simulink model "CACC_system_struct"  (Simulink 8.2)
settings: Solver=ode1  SolverMode=SingleTasking  StartTime=0.0  StopTime=inf  FixedStep=0.01  RelTol=1e-3
PreLoadFcn:
  | numd_dvsp = [0.3579 0 -0.3579];
  | dend_dvsp = [1 -1.846 0.8535];
  | simpleacc_param
PostLoadFcn:
  | , if any(exist('dsrtsu_mdlpostloadfcn', 'file') == [2, 3, 6]), try dsrtsu_mdlpostloadfcn('Execute', bdroot); catch fprintf('Error in PostLoadFcn (dsrtsu_mdlpostloadfcn) for model "%s":\n %s\n', bdroot, lasterr); end, end,
undefined symbols (not defined in the file or in its folder): command_mode, max_accel_m_s2, override_enabled, speed_command_m_s, wrench_effort_command
libraries: carma_platform x3, dsrc_transmitter x2, rtitttasklib x2, lightbar x2, srx_platform x1
(part 2 of 4)

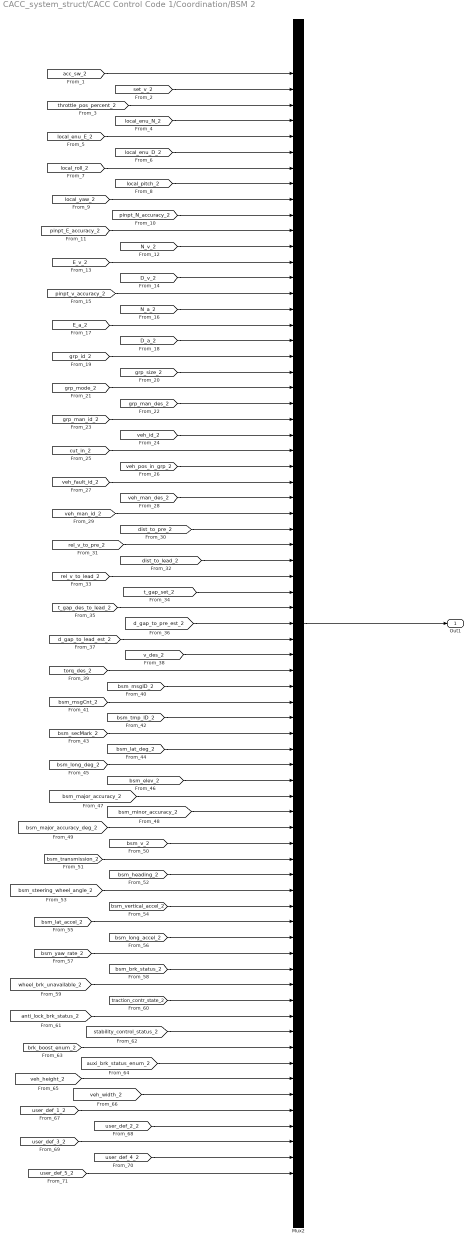
== system CACC_system_struct/CACC Control Code 1/Coordination/BSM 2 ==
  Mux2 : Mux  Inputs=71
  Out1 : Outport
  wires:
  Mux2/1 -> Out1/1
  [user_def_5_2] -> Mux2/71
  [user_def_4_2] -> Mux2/70
  [user_def_3_2] -> Mux2/69
  [user_def_2_2] -> Mux2/68
  [user_def_1_2] -> Mux2/67
  [brk_boost_enum_2] -> Mux2/63
  [auxi_brk_status_enum_2] -> Mux2/64
  [veh_width_2] -> Mux2/66
  [veh_height_2] -> Mux2/65
  [stability_control_status_2] -> Mux2/62
  [anti_lock_brk_status_2] -> Mux2/61
  [traction_contr_state_2] -> Mux2/60
  [wheel_brk_unavailable_2] -> Mux2/59
  [bsm_brk_status_2] -> Mux2/58
  [bsm_yaw_rate_2] -> Mux2/57
  [bsm_long_accel_2] -> Mux2/56
  [bsm_lat_accel_2] -> Mux2/55
  [bsm_vertical_accel_2] -> Mux2/54
  [bsm_steering_wheel_angle_2] -> Mux2/53
  [bsm_heading_2] -> Mux2/52
  [bsm_transmission_2] -> Mux2/51
  [bsm_v_2] -> Mux2/50
  [bsm_major_accuracy_deg_2] -> Mux2/49
  [bsm_minor_accuracy_2] -> Mux2/48
  [bsm_major_accuracy_2] -> Mux2/47
  [bsm_elev_2] -> Mux2/46
  [bsm_long_deg_2] -> Mux2/45
  [bsm_lat_deg_2] -> Mux2/44
  [bsm_secMark_2] -> Mux2/43
  [bsm_tmp_ID_2] -> Mux2/42
  [bsm_msgCnt_2] -> Mux2/41
  [bsm_msgID_2] -> Mux2/40
  [torq_des_2] -> Mux2/39
  [v_des_2] -> Mux2/38
  [d_gap_to_lead_est_2] -> Mux2/37
  [d_gap_to_pre_est_2] -> Mux2/36
  [t_gap_des_to_lead_2] -> Mux2/35
  [t_gap_set_2] -> Mux2/34
  [rel_v_to_lead_2] -> Mux2/33
  [dist_to_lead_2] -> Mux2/32
  [rel_v_to_pre_2] -> Mux2/31
  [dist_to_pre_2] -> Mux2/30
  [veh_man_id_2] -> Mux2/29
  [veh_man_des_2] -> Mux2/28
  [veh_fault_id_2] -> Mux2/27
  [veh_pos_in_grp_2] -> Mux2/26
  [acc_sw_2] -> Mux2/1
  [set_v_2] -> Mux2/2
  [throttle_pos_percent_2] -> Mux2/3
  [local_enu_N_2] -> Mux2/4
  [local_enu_E_2] -> Mux2/5
  [local_enu_D_2] -> Mux2/6
  [local_roll_2] -> Mux2/7
  [local_pitch_2] -> Mux2/8
  [local_yaw_2] -> Mux2/9
  [pinpt_N_accuracy_2] -> Mux2/10
  [pinpt_E_accuracy_2] -> Mux2/11
  [N_v_2] -> Mux2/12
  [E_v_2] -> Mux2/13
  [D_v_2] -> Mux2/14
  [pinpt_v_accuracy_2] -> Mux2/15
  [N_a_2] -> Mux2/16
  [E_a_2] -> Mux2/17
  [D_a_2] -> Mux2/18
  [grp_id_2] -> Mux2/19
  [grp_size_2] -> Mux2/20
  [grp_mode_2] -> Mux2/21
  [grp_man_des_2] -> Mux2/22
  [grp_man_id_2] -> Mux2/23
  [veh_id_2] -> Mux2/24
  [cut_in_2] -> Mux2/25

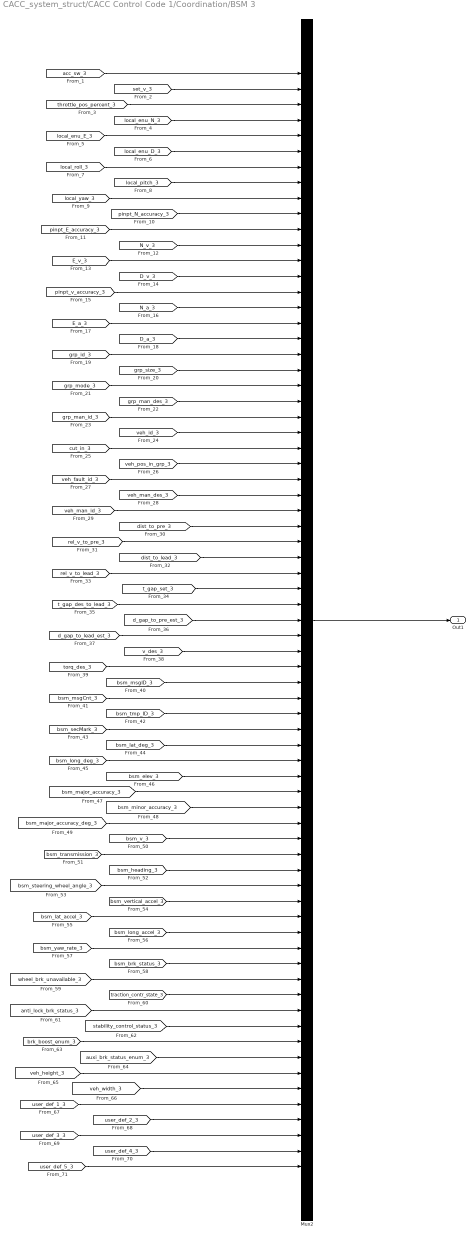
== system CACC_system_struct/CACC Control Code 1/Coordination/BSM 3 ==
  Mux2 : Mux  Inputs=71
  Out1 : Outport
  wires:
  Mux2/1 -> Out1/1
  [user_def_5_3] -> Mux2/71
  [user_def_4_3] -> Mux2/70
  [user_def_3_3] -> Mux2/69
  [user_def_2_3] -> Mux2/68
  [user_def_1_3] -> Mux2/67
  [brk_boost_enum_3] -> Mux2/63
  [auxi_brk_status_enum_3] -> Mux2/64
  [veh_width_3] -> Mux2/66
  [veh_height_3] -> Mux2/65
  [stability_control_status_3] -> Mux2/62
  [anti_lock_brk_status_3] -> Mux2/61
  [traction_contr_state_3] -> Mux2/60
  [wheel_brk_unavailable_3] -> Mux2/59
  [bsm_brk_status_3] -> Mux2/58
  [bsm_yaw_rate_3] -> Mux2/57
  [bsm_long_accel_3] -> Mux2/56
  [bsm_lat_accel_3] -> Mux2/55
  [bsm_vertical_accel_3] -> Mux2/54
  [bsm_steering_wheel_angle_3] -> Mux2/53
  [bsm_heading_3] -> Mux2/52
  [bsm_transmission_3] -> Mux2/51
  [bsm_v_3] -> Mux2/50
  [bsm_major_accuracy_deg_3] -> Mux2/49
  [bsm_minor_accuracy_3] -> Mux2/48
  [bsm_major_accuracy_3] -> Mux2/47
  [bsm_elev_3] -> Mux2/46
  [bsm_long_deg_3] -> Mux2/45
  [bsm_lat_deg_3] -> Mux2/44
  [bsm_secMark_3] -> Mux2/43
  [bsm_tmp_ID_3] -> Mux2/42
  [bsm_msgCnt_3] -> Mux2/41
  [bsm_msgID_3] -> Mux2/40
  [torq_des_3] -> Mux2/39
  [v_des_3] -> Mux2/38
  [d_gap_to_lead_est_3] -> Mux2/37
  [d_gap_to_pre_est_3] -> Mux2/36
  [t_gap_des_to_lead_3] -> Mux2/35
  [t_gap_set_3] -> Mux2/34
  [rel_v_to_lead_3] -> Mux2/33
  [dist_to_lead_3] -> Mux2/32
  [rel_v_to_pre_3] -> Mux2/31
  [dist_to_pre_3] -> Mux2/30
  [veh_man_id_3] -> Mux2/29
  [veh_man_des_3] -> Mux2/28
  [veh_fault_id_3] -> Mux2/27
  [veh_pos_in_grp_3] -> Mux2/26
  [acc_sw_3] -> Mux2/1
  [set_v_3] -> Mux2/2
  [throttle_pos_percent_3] -> Mux2/3
  [local_enu_N_3] -> Mux2/4
  [local_enu_E_3] -> Mux2/5
  [local_enu_D_3] -> Mux2/6
  [local_roll_3] -> Mux2/7
  [local_pitch_3] -> Mux2/8
  [local_yaw_3] -> Mux2/9
  [pinpt_N_accuracy_3] -> Mux2/10
  [pinpt_E_accuracy_3] -> Mux2/11
  [N_v_3] -> Mux2/12
  [E_v_3] -> Mux2/13
  [D_v_3] -> Mux2/14
  [pinpt_v_accuracy_3] -> Mux2/15
  [N_a_3] -> Mux2/16
  [E_a_3] -> Mux2/17
  [D_a_3] -> Mux2/18
  [grp_id_3] -> Mux2/19
  [grp_size_3] -> Mux2/20
  [grp_mode_3] -> Mux2/21
  [grp_man_des_3] -> Mux2/22
  [grp_man_id_3] -> Mux2/23
  [veh_id_3] -> Mux2/24
  [cut_in_3] -> Mux2/25

== system CACC_system_struct/CACC Control Code 1/Coordination/BSM 4 ==
  Mux2 : Mux  Inputs=71
  Out1 : Outport
  wires:
  Mux2/1 -> Out1/1
  [user_def_5_4] -> Mux2/71
  [user_def_4_4] -> Mux2/70
  [user_def_3_4] -> Mux2/69
  [user_def_2_4] -> Mux2/68
  [user_def_1_4] -> Mux2/67
  [brk_boost_enum_4] -> Mux2/63
  [auxi_brk_status_enum_4] -> Mux2/64
  [veh_width_4] -> Mux2/66
  [veh_height_4] -> Mux2/65
  [stability_control_status_4] -> Mux2/62
  [anti_lock_brk_status_4] -> Mux2/61
  [traction_contr_state_4] -> Mux2/60
  [wheel_brk_unavailable_4] -> Mux2/59
  [bsm_brk_status_4] -> Mux2/58
  [bsm_yaw_rate_4] -> Mux2/57
  [bsm_long_accel_4] -> Mux2/56
  [bsm_lat_accel_4] -> Mux2/55
  [bsm_vertical_accel_4] -> Mux2/54
  [bsm_steering_wheel_angle_4] -> Mux2/53
  [bsm_heading_4] -> Mux2/52
  [bsm_transmission_4] -> Mux2/51
  [bsm_v_4] -> Mux2/50
  [bsm_major_accuracy_deg_4] -> Mux2/49
  [bsm_minor_accuracy_4] -> Mux2/48
  [bsm_major_accuracy_4] -> Mux2/47
  [bsm_elev_4] -> Mux2/46
  [bsm_long_deg_4] -> Mux2/45
  [bsm_lat_deg_4] -> Mux2/44
  [bsm_secMark_4] -> Mux2/43
  [bsm_tmp_ID_4] -> Mux2/42
  [bsm_msgCnt_4] -> Mux2/41
  [bsm_msgID_4] -> Mux2/40
  [torq_des_4] -> Mux2/39
  [v_des_4] -> Mux2/38
  [d_gap_to_lead_est_4] -> Mux2/37
  [d_gap_to_pre_est_4] -> Mux2/36
  [t_gap_des_to_lead_4] -> Mux2/35
  [t_gap_set_4] -> Mux2/34
  [rel_v_to_lead_4] -> Mux2/33
  [dist_to_lead_4] -> Mux2/32
  [rel_v_to_pre_4] -> Mux2/31
  [dist_to_pre_4] -> Mux2/30
  [veh_man_id_4] -> Mux2/29
  [veh_man_des_4] -> Mux2/28
  [veh_fault_id_4] -> Mux2/27
  [veh_pos_in_grp_4] -> Mux2/26
  [acc_sw_4] -> Mux2/1
  [set_v_4] -> Mux2/2
  [throttle_pos_percent_4] -> Mux2/3
  [local_enu_N_4] -> Mux2/4
  [local_enu_E_4] -> Mux2/5
  [local_enu_D_4] -> Mux2/6
  [local_roll_4] -> Mux2/7
  [local_pitch_4] -> Mux2/8
  [local_yaw_4] -> Mux2/9
  [pinpt_N_accuracy_4] -> Mux2/10
  [pinpt_E_accuracy_4] -> Mux2/11
  [N_v_4] -> Mux2/12
  [E_v_4] -> Mux2/13
  [D_v_4] -> Mux2/14
  [pinpt_v_accuracy_4] -> Mux2/15
  [N_a_4] -> Mux2/16
  [E_a_4] -> Mux2/17
  [D_a_4] -> Mux2/18
  [grp_id_4] -> Mux2/19
  [grp_size_4] -> Mux2/20
  [grp_mode_4] -> Mux2/21
  [grp_man_des_4] -> Mux2/22
  [grp_man_id_4] -> Mux2/23
  [veh_id_4] -> Mux2/24
  [cut_in_4] -> Mux2/25

== system CACC_system_struct/CACC Control Code 1/Coordination/BSM 5 ==
  Mux2 : Mux  Inputs=71
  Out1 : Outport
  wires:
  Mux2/1 -> Out1/1
  [user_def_5_5] -> Mux2/71
  [user_def_4_5] -> Mux2/70
  [user_def_3_5] -> Mux2/69
  [user_def_2_5] -> Mux2/68
  [user_def_1_5] -> Mux2/67
  [brk_boost_enum_5] -> Mux2/63
  [auxi_brk_status_enum_5] -> Mux2/64
  [veh_width_5] -> Mux2/66
  [veh_height_5] -> Mux2/65
  [stability_control_status_5] -> Mux2/62
  [anti_lock_brk_status_5] -> Mux2/61
  [traction_contr_state_5] -> Mux2/60
  [wheel_brk_unavailable_5] -> Mux2/59
  [bsm_brk_status_5] -> Mux2/58
  [bsm_yaw_rate_5] -> Mux2/57
  [bsm_long_accel_5] -> Mux2/56
  [bsm_lat_accel_5] -> Mux2/55
  [bsm_vertical_accel_5] -> Mux2/54
  [bsm_steering_wheel_angle_5] -> Mux2/53
  [bsm_heading_5] -> Mux2/52
  [bsm_transmission_5] -> Mux2/51
  [bsm_v_5] -> Mux2/50
  [bsm_major_accuracy_deg_5] -> Mux2/49
  [bsm_minor_accuracy_5] -> Mux2/48
  [bsm_major_accuracy_5] -> Mux2/47
  [bsm_elev_5] -> Mux2/46
  [bsm_long_deg_5] -> Mux2/45
  [bsm_lat_deg_5] -> Mux2/44
  [bsm_secMark_5] -> Mux2/43
  [bsm_tmp_ID_5] -> Mux2/42
  [bsm_msgCnt_5] -> Mux2/41
  [bsm_msgID_5] -> Mux2/40
  [torq_des_5] -> Mux2/39
  [v_des_5] -> Mux2/38
  [d_gap_to_lead_est_5] -> Mux2/37
  [d_gap_to_pre_est_5] -> Mux2/36
  [t_gap_des_to_lead_5] -> Mux2/35
  [t_gap_set_5] -> Mux2/34
  [rel_v_to_lead_5] -> Mux2/33
  [dist_to_lead_5] -> Mux2/32
  [rel_v_to_pre_5] -> Mux2/31
  [dist_to_pre_5] -> Mux2/30
  [veh_man_id_5] -> Mux2/29
  [veh_man_des_5] -> Mux2/28
  [veh_fault_id_5] -> Mux2/27
  [veh_pos_in_grp_5] -> Mux2/26
  [acc_sw_5] -> Mux2/1
  [set_v_5] -> Mux2/2
  [throttle_pos_percent_5] -> Mux2/3
  [local_enu_N_5] -> Mux2/4
  [local_enu_E_5] -> Mux2/5
  [local_enu_D_5] -> Mux2/6
  [local_roll_5] -> Mux2/7
  [local_pitch_5] -> Mux2/8
  [local_yaw_5] -> Mux2/9
  [pinpt_N_accuracy_5] -> Mux2/10
  [pinpt_E_accuracy_5] -> Mux2/11
  [N_v_5] -> Mux2/12
  [E_v_5] -> Mux2/13
  [D_v_5] -> Mux2/14
  [pinpt_v_accuracy_5] -> Mux2/15
  [N_a_5] -> Mux2/16
  [E_a_5] -> Mux2/17
  [D_a_5] -> Mux2/18
  [grp_id_5] -> Mux2/19
  [grp_size_5] -> Mux2/20
  [grp_mode_5] -> Mux2/21
  [grp_man_des_5] -> Mux2/22
  [grp_man_id_5] -> Mux2/23
  [veh_id_5] -> Mux2/24
  [cut_in_5] -> Mux2/25

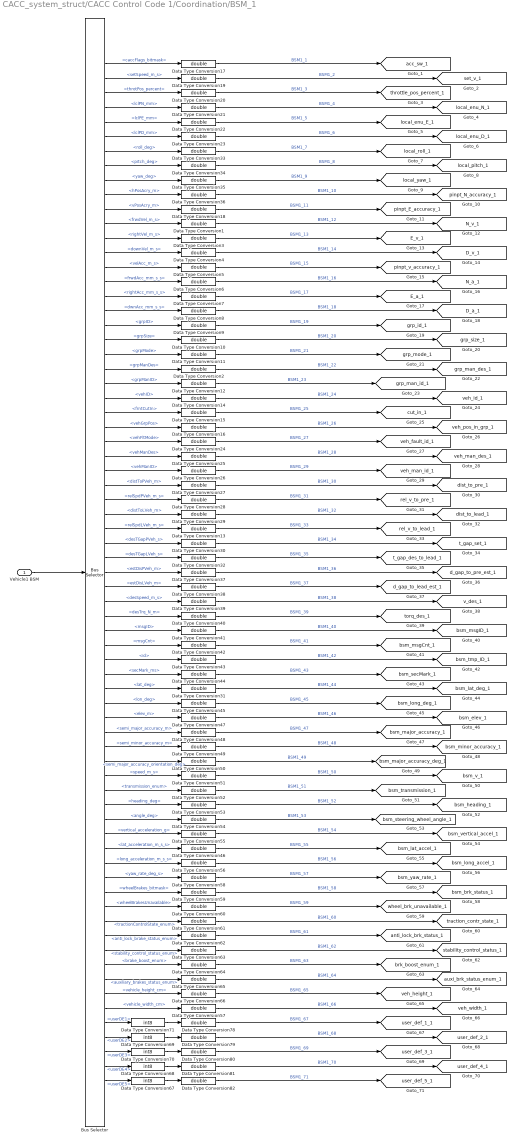
== system CACC_system_struct/CACC Control Code 1/Coordination/BSM_1 ==
  Vehicle1 BSM : Inport
  Bus Selector : BusSelector  OutputSignals=caccFlags_bitmask,setSpeed_m_s,throtPos_percent,lclPN_mm,lclPE_mm,lclPD_mm,roll_deg,pitch_deg,yaw_deg,hPosAcry_m,vPosAcry_m,frwdVel_m_s,rightVel_m_s,downVel_m_s,velAcc_m_s,frwdAcc_mm_s_s,rightAcc_mm_s_s,dwnAcc_mm_s_s,grpID,grpSize,grpMode,grpManDes,grpManID,vehID,frntCutIn,vehGrpPos,vehFltMode,vehManDes,vehManID,distToPVeh_m,relSpdPVeh_m_s,distToLVeh_m,relSpdLVeh_m_s,desTGapPVeh_s,desTGapLVeh_s,estDisPVeh_m,estDisLVeh_m,desSpeed_m_s,desTrq_N_m,msgID,msgCnt,id,secMark_ms,lat_deg,lon_deg,elev_m,semi_major_accuracy_m,semi_minor_accuracy_m,semi_major_accuracy_orientation_deg,speed_m_s,transmission_enum,heading_deg,angle_deg,vertical_acceleration_g,lat_acceleration_m_s_s,long_acceleration_m_s_s,yaw_rate_deg_s,wheelBrakes_bitmask,wheelBrakesUnavailable,tractionControlState_enum,anti_lock_brake_status_enum,stability_control_status_enum,brake_boost_enum,auxiliary_brakes_status_enum,vehicle_height_cm,vehicle_width_cm,userDE1,userDE2,userDE3,userDE4,userDE5
  Data Type Conversion{1..66,78..82} (71 alike) : DataTypeConversion  OutMin=[0]  OutMax=[5]  OutDataTypeStr=double
  Data Type Conversion{67..71} (5 alike) : DataTypeConversion  OutMin=[-128]  OutMax=[127]  OutDataTypeStr=int8  ConvertRealWorld=Stored Integer (SI)
  tag scope: D_a_1=global, D_v_1=global, E_a_1=global, E_v_1=global, N_a_1=global, N_v_1=global, acc_sw_1=global, anti_lock_brk_status_1=global, auxi_brk_status_enum_1=global, brk_boost_enum_1=global, bsm_brk_status_1=global, bsm_elev_1=global, bsm_heading_1=global, bsm_lat_accel_1=global, bsm_lat_deg_1=global, bsm_long_accel_1=global, bsm_long_deg_1=global, bsm_major_accuracy_1=global, bsm_major_accuracy_deg_1=global, bsm_minor_accuracy_1=global, bsm_msgCnt_1=global, bsm_msgID_1=global, bsm_secMark_1=global, bsm_steering_wheel_angle_1=global, bsm_tmp_ID_1=global, bsm_transmission_1=global, bsm_v_1=global, bsm_vertical_accel_1=global, bsm_yaw_rate_1=global, cut_in_1=global, d_gap_to_lead_est_1=global, d_gap_to_pre_est_1=global, dist_to_lead_1=global, dist_to_pre_1=global, grp_id_1=global, grp_man_des_1=global, grp_man_id_1=global, grp_mode_1=global, grp_size_1=global, local_enu_D_1=global, local_enu_E_1=global, local_enu_N_1=global, local_pitch_1=global, local_roll_1=global, local_yaw_1=global, pinpt_E_accuracy_1=global, pinpt_N_accuracy_1=global, pinpt_v_accuracy_1=global, rel_v_to_lead_1=global, rel_v_to_pre_1=global, set_v_1=global, stability_control_status_1=global, t_gap_des_to_lead_1=global, t_gap_set_1=global, throttle_pos_percent_1=global, torq_des_1=global, traction_contr_state_1=global, user_def_1_1=global, user_def_2_1=global, user_def_3_1=global, user_def_4_1=global, user_def_5_1=global, v_des_1=global, veh_fault_id_1=global, veh_height_1=global, veh_id_1=global, veh_man_des_1=global, veh_man_id_1=global, veh_pos_in_grp_1=global, veh_width_1=global, wheel_brk_unavailable_1=global
  wires:
  Vehicle1 BSM/1 -> Bus Selector/1
  Bus Selector/34 -> Data Type Conversion30/1  "<desTGapPVeh_s>"
  Bus Selector/33 -> Data Type Conversion13/1  "<relSpdLVeh_m_s>"
  Bus Selector/2 -> Data Type Conversion19/1  "<setSpeed_m_s>"
  Bus Selector/1 -> Data Type Conversion17/1  "<caccFlags_bitmask>"
  Bus Selector/7 -> Data Type Conversion33/1  "<roll_deg>"
  Bus Selector/3 -> Data Type Conversion20/1  "<throtPos_percent>"
  Bus Selector/9 -> Data Type Conversion35/1  "<yaw_deg>"
  Bus Selector/8 -> Data Type Conversion34/1  "<pitch_deg>"
  Bus Selector/11 -> Data Type Conversion18/1  "<vPosAcry_m>"
  Bus Selector/10 -> Data Type Conversion36/1  "<hPosAcry_m>"
  Bus Selector/13 -> Data Type Conversion3/1  "<rightVel_m_s>"
  Bus Selector/12 -> Data Type Conversion1/1  "<frwdVel_m_s>"
  Bus Selector/15 -> Data Type Conversion5/1  "<velAcc_m_s>"
  Bus Selector/14 -> Data Type Conversion4/1  "<downVel_m_s>"
  Bus Selector/17 -> Data Type Conversion7/1  "<rightAcc_mm_s_s>"
  Bus Selector/16 -> Data Type Conversion6/1  "<frwdAcc_mm_s_s>"
  Bus Selector/19 -> Data Type Conversion9/1  "<grpID>"
  Bus Selector/18 -> Data Type Conversion8/1  "<dwnAcc_mm_s_s>"
  Bus Selector/21 -> Data Type Conversion11/1  "<grpMode>"
  Bus Selector/20 -> Data Type Conversion10/1  "<grpSize>"
  Bus Selector/22 -> Data Type Conversion2/1  "<grpManDes>"
  Bus Selector/25 -> Data Type Conversion15/1  "<frntCutIn>"
  Bus Selector/24 -> Data Type Conversion14/1  "<vehID>"
  Bus Selector/27 -> Data Type Conversion24/1  "<vehFltMode>"
  Bus Selector/26 -> Data Type Conversion16/1  "<vehGrpPos>"
  Bus Selector/30 -> Data Type Conversion27/1  "<distToPVeh_m>"
  Bus Selector/29 -> Data Type Conversion26/1  "<vehManID>"
  Bus Selector/32 -> Data Type Conversion29/1  "<distToLVeh_m>"
  Bus Selector/36 -> Data Type Conversion37/1  "<estDisPVeh_m>"
  Bus Selector/35 -> Data Type Conversion32/1  "<desTGapLVeh_s>"
  Bus Selector/38 -> Data Type Conversion39/1  "<desSpeed_m_s>"
  Bus Selector/37 -> Data Type Conversion38/1  "<estDisLVeh_m>"
  Bus Selector/40 -> Data Type Conversion41/1  "<msgID>"
  Bus Selector/39 -> Data Type Conversion40/1  "<desTrq_N_m>"
  Bus Selector/42 -> Data Type Conversion43/1  "<id>"
  Bus Selector/41 -> Data Type Conversion42/1  "<msgCnt>"
  Bus Selector/44 -> Data Type Conversion31/1  "<lat_deg>"
  Bus Selector/43 -> Data Type Conversion44/1  "<secMark_ms>"
  Bus Selector/46 -> Data Type Conversion47/1  "<elev_m>"
  Bus Selector/45 -> Data Type Conversion45/1  "<lon_deg>"
  Bus Selector/48 -> Data Type Conversion49/1  "<semi_minor_accuracy_m>"
  Bus Selector/47 -> Data Type Conversion48/1  "<semi_major_accuracy_m>"
  Bus Selector/50 -> Data Type Conversion51/1  "<speed_m_s>"
  Bus Selector/49 -> Data Type Conversion50/1  "<semi_major_accuracy_orientation_deg>"
  Bus Selector/52 -> Data Type Conversion53/1  "<heading_deg>"
  Bus Selector/51 -> Data Type Conversion52/1  "<transmission_enum>"
  Bus Selector/54 -> Data Type Conversion55/1  "<vertical_acceleration_g>"
  Bus Selector/53 -> Data Type Conversion54/1  "<angle_deg>"
  Bus Selector/56 -> Data Type Conversion56/1  "<long_acceleration_m_s_s>"
  Bus Selector/55 -> Data Type Conversion46/1  "<lat_acceleration_m_s_s>"
  Bus Selector/58 -> Data Type Conversion59/1  "<wheelBrakes_bitmask>"
  Bus Selector/57 -> Data Type Conversion58/1  "<yaw_rate_deg_s>"
  Bus Selector/60 -> Data Type Conversion61/1  "<tractionControlState_enum>"
  Bus Selector/59 -> Data Type Conversion60/1  "<wheelBrakesUnavailable>"
  Bus Selector/62 -> Data Type Conversion63/1  "<stability_control_status_enum>"
  Bus Selector/61 -> Data Type Conversion62/1  "<anti_lock_brake_status_enum>"
  Bus Selector/64 -> Data Type Conversion65/1  "<auxiliary_brakes_status_enum>"
  Bus Selector/63 -> Data Type Conversion64/1  "<brake_boost_enum>"
  Bus Selector/66 -> Data Type Conversion57/1  "<vehicle_width_cm>"
  Bus Selector/65 -> Data Type Conversion66/1  "<vehicle_height_cm>"
  Bus Selector/4 -> Data Type Conversion21/1  "<lclPN_mm>"
  Bus Selector/5 -> Data Type Conversion22/1  "<lclPE_mm>"
  Bus Selector/6 -> Data Type Conversion23/1  "<lclPD_mm>"
  Bus Selector/23 -> Data Type Conversion12/1  "<grpManID>"
  Bus Selector/28 -> Data Type Conversion25/1  "<vehManDes>"
  Bus Selector/31 -> Data Type Conversion28/1  "<relSpdPVeh_m_s>"
  Bus Selector/67 -> Data Type Conversion71/1  "<userDE1>"
  Bus Selector/68 -> Data Type Conversion69/1  "<userDE2>"
  Bus Selector/69 -> Data Type Conversion70/1  "<userDE3>"
  Bus Selector/70 -> Data Type Conversion68/1  "<userDE4>"
  Bus Selector/71 -> Data Type Conversion67/1  "<userDE5>"
  Data Type Conversion25/1 -> [veh_man_des_1]  "BSM1_28"
  Data Type Conversion17/1 -> [acc_sw_1]  "BSM1_1"
  Data Type Conversion52/1 -> [bsm_transmission_1]  "BSM1_51"
  Data Type Conversion1/1 -> [N_v_1]  "BSM1_12"
  Data Type Conversion11/1 -> [grp_mode_1]  "BSM1_21"
  Data Type Conversion13/1 -> [rel_v_to_lead_1]  "BSM1_33"
  Data Type Conversion3/1 -> [E_v_1]  "BSM1_13"
  Data Type Conversion56/1 -> [bsm_long_accel_1]  "BSM1_56"
  Data Type Conversion14/1 -> [veh_id_1]  "BSM1_24"
  Data Type Conversion18/1 -> [pinpt_E_accuracy_1]  "BSM1_11"
  Data Type Conversion53/1 -> [bsm_heading_1]  "BSM1_52"
  Data Type Conversion55/1 -> [bsm_vertical_accel_1]  "BSM1_54"
  Data Type Conversion27/1 -> [dist_to_pre_1]  "BSM1_30"
  Data Type Conversion23/1 -> [local_enu_D_1]  "BSM1_6"
  Data Type Conversion21/1 -> [local_enu_N_1]  "BSM1_4"
  Data Type Conversion22/1 -> [local_enu_E_1]  "BSM1_5"
  Data Type Conversion28/1 -> [rel_v_to_pre_1]  "BSM1_31"
  Data Type Conversion12/1 -> [grp_man_id_1]  "BSM1_23"
  Data Type Conversion49/1 -> [bsm_minor_accuracy_1]  "BSM1_48"
  Data Type Conversion24/1 -> [veh_fault_id_1]  "BSM1_27"
  Data Type Conversion26/1 -> [veh_man_id_1]  "BSM1_29"
  Data Type Conversion10/1 -> [grp_size_1]  "BSM1_20"
  Data Type Conversion19/1 -> [set_v_1]  "BSM1_2"
  Data Type Conversion29/1 -> [dist_to_lead_1]  "BSM1_32"
  Data Type Conversion51/1 -> [bsm_v_1]  "BSM1_50"
  Data Type Conversion57/1 -> [veh_width_1]  "BSM1_66"
  Data Type Conversion20/1 -> [throttle_pos_percent_1]  "BSM1_3"
  Data Type Conversion2/1 -> [grp_man_des_1]  "BSM1_22"
  Data Type Conversion5/1 -> [pinpt_v_accuracy_1]  "BSM1_15"
  Data Type Conversion54/1 -> [bsm_steering_wheel_angle_1]  "BSM1_53"
  Data Type Conversion50/1 -> [bsm_major_accuracy_deg_1]  "BSM1_49"
  Data Type Conversion16/1 -> [veh_pos_in_grp_1]  "BSM1_26"
  Data Type Conversion15/1 -> [cut_in_1]  "BSM1_25"
  Data Type Conversion48/1 -> [bsm_major_accuracy_1]  "BSM1_47"
  Data Type Conversion47/1 -> [bsm_elev_1]  "BSM1_46"
  Data Type Conversion46/1 -> [bsm_lat_accel_1]  "BSM1_55"
  Data Type Conversion45/1 -> [bsm_long_deg_1]  "BSM1_45"
  Data Type Conversion44/1 -> [bsm_secMark_1]  "BSM1_43"
  Data Type Conversion43/1 -> [bsm_tmp_ID_1]  "BSM1_42"
  Data Type Conversion42/1 -> [bsm_msgCnt_1]  "BSM1_41"
  Data Type Conversion41/1 -> [bsm_msgID_1]  "BSM1_40"
  Data Type Conversion40/1 -> [torq_des_1]  "BSM1_39"
  Data Type Conversion4/1 -> [D_v_1]  "BSM1_14"
  Data Type Conversion39/1 -> [v_des_1]  "BSM1_38"
  Data Type Conversion37/1 -> [d_gap_to_pre_est_1]  "BSM1_36"
  Data Type Conversion38/1 -> [d_gap_to_lead_est_1]  "BSM1_37"
  Data Type Conversion35/1 -> [local_yaw_1]  "BSM1_9"
  Data Type Conversion33/1 -> [local_roll_1]  "BSM1_7"
  Data Type Conversion30/1 -> [t_gap_set_1]  "BSM1_34"
  Data Type Conversion36/1 -> [pinpt_N_accuracy_1]  "BSM1_10"
  Data Type Conversion34/1 -> [local_pitch_1]  "BSM1_8"
  Data Type Conversion32/1 -> [t_gap_des_to_lead_1]  "BSM1_35"
  Data Type Conversion31/1 -> [bsm_lat_deg_1]  "BSM1_44"
  Data Type Conversion58/1 -> [bsm_yaw_rate_1]  "BSM1_57"
  Data Type Conversion59/1 -> [bsm_brk_status_1]  "BSM1_58"
  Data Type Conversion6/1 -> [N_a_1]  "BSM1_16"
  Data Type Conversion60/1 -> [wheel_brk_unavailable_1]  "BSM1_59"
  Data Type Conversion61/1 -> [traction_contr_state_1]  "BSM1_60"
  Data Type Conversion62/1 -> [anti_lock_brk_status_1]  "BSM1_61"
  Data Type Conversion63/1 -> [stability_control_status_1]  "BSM1_62"
  Data Type Conversion64/1 -> [brk_boost_enum_1]  "BSM1_63"
  Data Type Conversion65/1 -> [auxi_brk_status_enum_1]  "BSM1_64"
  Data Type Conversion66/1 -> [veh_height_1]  "BSM1_65"
  Data Type Conversion7/1 -> [E_a_1]  "BSM1_17"
  Data Type Conversion78/1 -> [user_def_1_1]  "BSM1_67"
  Data Type Conversion79/1 -> [user_def_2_1]  "BSM1_68"
  Data Type Conversion8/1 -> [D_a_1]  "BSM1_18"
  Data Type Conversion80/1 -> [user_def_3_1]  "BSM1_69"
  Data Type Conversion81/1 -> [user_def_4_1]  "BSM1_70"
  Data Type Conversion82/1 -> [user_def_5_1]  "BSM1_71"
  Data Type Conversion9/1 -> [grp_id_1]  "BSM1_19"
  Data Type Conversion67/1 -> Data Type Conversion82/1
  Data Type Conversion68/1 -> Data Type Conversion81/1
  Data Type Conversion70/1 -> Data Type Conversion80/1
  Data Type Conversion69/1 -> Data Type Conversion79/1
  Data Type Conversion71/1 -> Data Type Conversion78/1

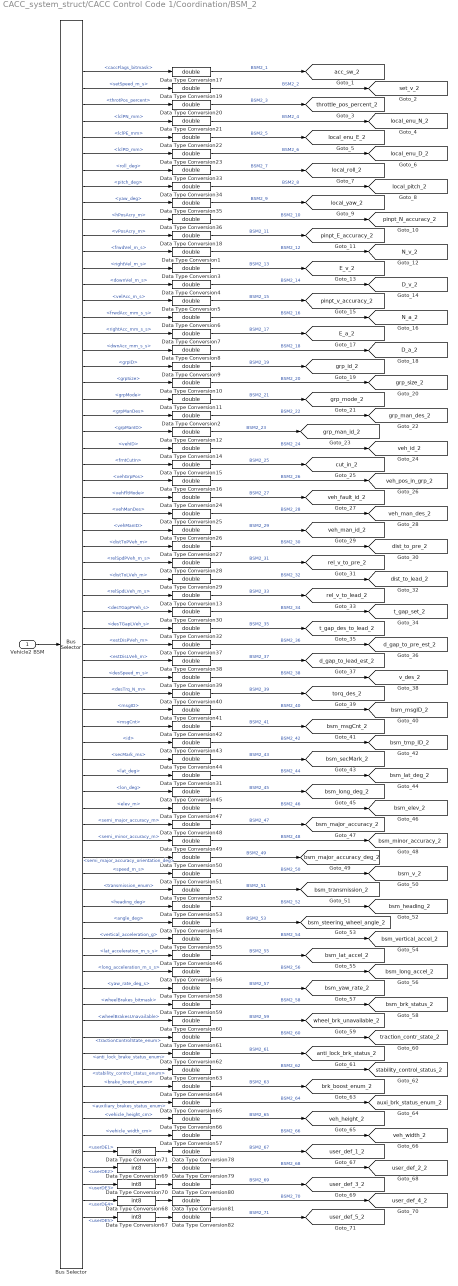
== system CACC_system_struct/CACC Control Code 1/Coordination/BSM_2 ==
  Vehicle2 BSM : Inport
  Bus Selector : BusSelector  OutputSignals=caccFlags_bitmask,setSpeed_m_s,throtPos_percent,lclPN_mm,lclPE_mm,lclPD_mm,roll_deg,pitch_deg,yaw_deg,hPosAcry_m,vPosAcry_m,frwdVel_m_s,rightVel_m_s,downVel_m_s,velAcc_m_s,frwdAcc_mm_s_s,rightAcc_mm_s_s,dwnAcc_mm_s_s,grpID,grpSize,grpMode,grpManDes,grpManID,vehID,frntCutIn,vehGrpPos,vehFltMode,vehManDes,vehManID,distToPVeh_m,relSpdPVeh_m_s,distToLVeh_m,relSpdLVeh_m_s,desTGapPVeh_s,desTGapLVeh_s,estDisPVeh_m,estDisLVeh_m,desSpeed_m_s,desTrq_N_m,msgID,msgCnt,id,secMark_ms,lat_deg,lon_deg,elev_m,semi_major_accuracy_m,semi_minor_accuracy_m,semi_major_accuracy_orientation_deg,speed_m_s,transmission_enum,heading_deg,angle_deg,vertical_acceleration_g,lat_acceleration_m_s_s,long_acceleration_m_s_s,yaw_rate_deg_s,wheelBrakes_bitmask,wheelBrakesUnavailable,tractionControlState_enum,anti_lock_brake_status_enum,stability_control_status_enum,brake_boost_enum,auxiliary_brakes_status_enum,vehicle_height_cm,vehicle_width_cm,userDE1,userDE2,userDE3,userDE4,userDE5
  Data Type Conversion{1..66,78..82} (71 alike) : DataTypeConversion  OutMin=[0]  OutMax=[5]  OutDataTypeStr=double
  Data Type Conversion{67..71} (5 alike) : DataTypeConversion  OutMin=[-128]  OutMax=[127]  OutDataTypeStr=int8  ConvertRealWorld=Stored Integer (SI)
  tag scope: D_a_2=global, D_v_2=global, E_a_2=global, E_v_2=global, N_a_2=global, N_v_2=global, acc_sw_2=global, anti_lock_brk_status_2=global, auxi_brk_status_enum_2=global, brk_boost_enum_2=global, bsm_brk_status_2=global, bsm_elev_2=global, bsm_heading_2=global, bsm_lat_accel_2=global, bsm_lat_deg_2=global, bsm_long_accel_2=global, bsm_long_deg_2=global, bsm_major_accuracy_2=global, bsm_major_accuracy_deg_2=global, bsm_minor_accuracy_2=global, bsm_msgCnt_2=global, bsm_msgID_2=global, bsm_secMark_2=global, bsm_steering_wheel_angle_2=global, bsm_tmp_ID_2=global, bsm_transmission_2=global, bsm_v_2=global, bsm_vertical_accel_2=global, bsm_yaw_rate_2=global, cut_in_2=global, d_gap_to_lead_est_2=global, d_gap_to_pre_est_2=global, dist_to_lead_2=global, dist_to_pre_2=global, grp_id_2=global, grp_man_des_2=global, grp_man_id_2=global, grp_mode_2=global, grp_size_2=global, local_enu_D_2=global, local_enu_E_2=global, local_enu_N_2=global, local_pitch_2=global, local_roll_2=global, local_yaw_2=global, pinpt_E_accuracy_2=global, pinpt_N_accuracy_2=global, pinpt_v_accuracy_2=global, rel_v_to_lead_2=global, rel_v_to_pre_2=global, set_v_2=global, stability_control_status_2=global, t_gap_des_to_lead_2=global, t_gap_set_2=global, throttle_pos_percent_2=global, torq_des_2=global, traction_contr_state_2=global, user_def_1_2=global, user_def_2_2=global, user_def_3_2=global, user_def_4_2=global, user_def_5_2=global, v_des_2=global, veh_fault_id_2=global, veh_height_2=global, veh_id_2=global, veh_man_des_2=global, veh_man_id_2=global, veh_pos_in_grp_2=global, veh_width_2=global, wheel_brk_unavailable_2=global
  wires:
  Vehicle2 BSM/1 -> Bus Selector/1
  Bus Selector/34 -> Data Type Conversion30/1  "<desTGapPVeh_s>"
  Bus Selector/33 -> Data Type Conversion13/1  "<relSpdLVeh_m_s>"
  Bus Selector/2 -> Data Type Conversion19/1  "<setSpeed_m_s>"
  Bus Selector/1 -> Data Type Conversion17/1  "<caccFlags_bitmask>"
  Bus Selector/7 -> Data Type Conversion33/1  "<roll_deg>"
  Bus Selector/3 -> Data Type Conversion20/1  "<throtPos_percent>"
  Bus Selector/9 -> Data Type Conversion35/1  "<yaw_deg>"
  Bus Selector/8 -> Data Type Conversion34/1  "<pitch_deg>"
  Bus Selector/11 -> Data Type Conversion18/1  "<vPosAcry_m>"
  Bus Selector/10 -> Data Type Conversion36/1  "<hPosAcry_m>"
  Bus Selector/13 -> Data Type Conversion3/1  "<rightVel_m_s>"
  Bus Selector/12 -> Data Type Conversion1/1  "<frwdVel_m_s>"
  Bus Selector/15 -> Data Type Conversion5/1  "<velAcc_m_s>"
  Bus Selector/14 -> Data Type Conversion4/1  "<downVel_m_s>"
  Bus Selector/17 -> Data Type Conversion7/1  "<rightAcc_mm_s_s>"
  Bus Selector/16 -> Data Type Conversion6/1  "<frwdAcc_mm_s_s>"
  Bus Selector/19 -> Data Type Conversion9/1  "<grpID>"
  Bus Selector/18 -> Data Type Conversion8/1  "<dwnAcc_mm_s_s>"
  Bus Selector/21 -> Data Type Conversion11/1  "<grpMode>"
  Bus Selector/20 -> Data Type Conversion10/1  "<grpSize>"
  Bus Selector/22 -> Data Type Conversion2/1  "<grpManDes>"
  Bus Selector/25 -> Data Type Conversion15/1  "<frntCutIn>"
  Bus Selector/24 -> Data Type Conversion14/1  "<vehID>"
  Bus Selector/27 -> Data Type Conversion24/1  "<vehFltMode>"
  Bus Selector/26 -> Data Type Conversion16/1  "<vehGrpPos>"
  Bus Selector/30 -> Data Type Conversion27/1  "<distToPVeh_m>"
  Bus Selector/29 -> Data Type Conversion26/1  "<vehManID>"
  Bus Selector/32 -> Data Type Conversion29/1  "<distToLVeh_m>"
  Bus Selector/36 -> Data Type Conversion37/1  "<estDisPVeh_m>"
  Bus Selector/35 -> Data Type Conversion32/1  "<desTGapLVeh_s>"
  Bus Selector/38 -> Data Type Conversion39/1  "<desSpeed_m_s>"
  Bus Selector/37 -> Data Type Conversion38/1  "<estDisLVeh_m>"
  Bus Selector/40 -> Data Type Conversion41/1  "<msgID>"
  Bus Selector/39 -> Data Type Conversion40/1  "<desTrq_N_m>"
  Bus Selector/42 -> Data Type Conversion43/1  "<id>"
  Bus Selector/41 -> Data Type Conversion42/1  "<msgCnt>"
  Bus Selector/44 -> Data Type Conversion31/1  "<lat_deg>"
  Bus Selector/43 -> Data Type Conversion44/1  "<secMark_ms>"
  Bus Selector/46 -> Data Type Conversion47/1  "<elev_m>"
  Bus Selector/45 -> Data Type Conversion45/1  "<lon_deg>"
  Bus Selector/48 -> Data Type Conversion49/1  "<semi_minor_accuracy_m>"
  Bus Selector/47 -> Data Type Conversion48/1  "<semi_major_accuracy_m>"
  Bus Selector/50 -> Data Type Conversion51/1  "<speed_m_s>"
  Bus Selector/49 -> Data Type Conversion50/1  "<semi_major_accuracy_orientation_deg>"
  Bus Selector/52 -> Data Type Conversion53/1  "<heading_deg>"
  Bus Selector/51 -> Data Type Conversion52/1  "<transmission_enum>"
  Bus Selector/54 -> Data Type Conversion55/1  "<vertical_acceleration_g>"
  Bus Selector/53 -> Data Type Conversion54/1  "<angle_deg>"
  Bus Selector/56 -> Data Type Conversion56/1  "<long_acceleration_m_s_s>"
  Bus Selector/55 -> Data Type Conversion46/1  "<lat_acceleration_m_s_s>"
  Bus Selector/58 -> Data Type Conversion59/1  "<wheelBrakes_bitmask>"
  Bus Selector/57 -> Data Type Conversion58/1  "<yaw_rate_deg_s>"
  Bus Selector/60 -> Data Type Conversion61/1  "<tractionControlState_enum>"
  Bus Selector/59 -> Data Type Conversion60/1  "<wheelBrakesUnavailable>"
  Bus Selector/62 -> Data Type Conversion63/1  "<stability_control_status_enum>"
  Bus Selector/61 -> Data Type Conversion62/1  "<anti_lock_brake_status_enum>"
  Bus Selector/64 -> Data Type Conversion65/1  "<auxiliary_brakes_status_enum>"
  Bus Selector/63 -> Data Type Conversion64/1  "<brake_boost_enum>"
  Bus Selector/66 -> Data Type Conversion57/1  "<vehicle_width_cm>"
  Bus Selector/65 -> Data Type Conversion66/1  "<vehicle_height_cm>"
  Bus Selector/4 -> Data Type Conversion21/1  "<lclPN_mm>"
  Bus Selector/5 -> Data Type Conversion22/1  "<lclPE_mm>"
  Bus Selector/6 -> Data Type Conversion23/1  "<lclPD_mm>"
  Bus Selector/23 -> Data Type Conversion12/1  "<grpManID>"
  Bus Selector/28 -> Data Type Conversion25/1  "<vehManDes>"
  Bus Selector/31 -> Data Type Conversion28/1  "<relSpdPVeh_m_s>"
  Bus Selector/67 -> Data Type Conversion71/1  "<userDE1>"
  Bus Selector/68 -> Data Type Conversion69/1  "<userDE2>"
  Bus Selector/69 -> Data Type Conversion70/1  "<userDE3>"
  Bus Selector/70 -> Data Type Conversion68/1  "<userDE4>"
  Bus Selector/71 -> Data Type Conversion67/1  "<userDE5>"
  Data Type Conversion10/1 -> [grp_size_2]  "BSM2_20"
  Data Type Conversion11/1 -> [grp_mode_2]  "BSM2_21"
  Data Type Conversion14/1 -> [veh_id_2]  "BSM2_24"
  Data Type Conversion20/1 -> [throttle_pos_percent_2]  "BSM2_3"
  Data Type Conversion21/1 -> [local_enu_N_2]  "BSM2_4"
  Data Type Conversion18/1 -> [pinpt_E_accuracy_2]  "BSM2_11"
  Data Type Conversion15/1 -> [cut_in_2]  "BSM2_25"
  Data Type Conversion17/1 -> [acc_sw_2]  "BSM2_1"
  Data Type Conversion13/1 -> [rel_v_to_lead_2]  "BSM2_33"
  Data Type Conversion16/1 -> [veh_pos_in_grp_2]  "BSM2_26"
  Data Type Conversion22/1 -> [local_enu_E_2]  "BSM2_5"
  Data Type Conversion2/1 -> [grp_man_des_2]  "BSM2_22"
  Data Type Conversion1/1 -> [N_v_2]  "BSM2_12"
  Data Type Conversion12/1 -> [grp_man_id_2]  "BSM2_23"
  Data Type Conversion23/1 -> [local_enu_D_2]  "BSM2_6"
  Data Type Conversion19/1 -> [set_v_2]  "BSM2_2"
  Data Type Conversion24/1 -> [veh_fault_id_2]  "BSM2_27"
  Data Type Conversion25/1 -> [veh_man_des_2]  "BSM2_28"
  Data Type Conversion26/1 -> [veh_man_id_2]  "BSM2_29"
  Data Type Conversion27/1 -> [dist_to_pre_2]  "BSM2_30"
  Data Type Conversion28/1 -> [rel_v_to_pre_2]  "BSM2_31"
  Data Type Conversion29/1 -> [dist_to_lead_2]  "BSM2_32"
  Data Type Conversion3/1 -> [E_v_2]  "BSM2_13"
  Data Type Conversion30/1 -> [t_gap_set_2]  "BSM2_34"
  Data Type Conversion31/1 -> [bsm_lat_deg_2]  "BSM2_44"
  Data Type Conversion32/1 -> [t_gap_des_to_lead_2]  "BSM2_35"
  Data Type Conversion33/1 -> [local_roll_2]  "BSM2_7"
  Data Type Conversion34/1 -> [local_pitch_2]  "BSM2_8"
  Data Type Conversion35/1 -> [local_yaw_2]  "BSM2_9"
  Data Type Conversion36/1 -> [pinpt_N_accuracy_2]  "BSM2_10"
  Data Type Conversion37/1 -> [d_gap_to_pre_est_2]  "BSM2_36"
  Data Type Conversion38/1 -> [d_gap_to_lead_est_2]  "BSM2_37"
  Data Type Conversion39/1 -> [v_des_2]  "BSM2_38"
  Data Type Conversion4/1 -> [D_v_2]  "BSM2_14"
  Data Type Conversion40/1 -> [torq_des_2]  "BSM2_39"
  Data Type Conversion41/1 -> [bsm_msgID_2]  "BSM2_40"
  Data Type Conversion42/1 -> [bsm_msgCnt_2]  "BSM2_41"
  Data Type Conversion43/1 -> [bsm_tmp_ID_2]  "BSM2_42"
  Data Type Conversion44/1 -> [bsm_secMark_2]  "BSM2_43"
  Data Type Conversion45/1 -> [bsm_long_deg_2]  "BSM2_45"
  Data Type Conversion46/1 -> [bsm_lat_accel_2]  "BSM2_55"
  Data Type Conversion47/1 -> [bsm_elev_2]  "BSM2_46"
  Data Type Conversion48/1 -> [bsm_major_accuracy_2]  "BSM2_47"
  Data Type Conversion49/1 -> [bsm_minor_accuracy_2]  "BSM2_48"
  Data Type Conversion5/1 -> [pinpt_v_accuracy_2]  "BSM2_15"
  Data Type Conversion50/1 -> [bsm_major_accuracy_deg_2]  "BSM2_49"
  Data Type Conversion51/1 -> [bsm_v_2]  "BSM2_50"
  Data Type Conversion52/1 -> [bsm_transmission_2]  "BSM2_51"
  Data Type Conversion53/1 -> [bsm_heading_2]  "BSM2_52"
  Data Type Conversion54/1 -> [bsm_steering_wheel_angle_2]  "BSM2_53"
  Data Type Conversion55/1 -> [bsm_vertical_accel_2]  "BSM2_54"
  Data Type Conversion56/1 -> [bsm_long_accel_2]  "BSM2_56"
  Data Type Conversion57/1 -> [veh_width_2]  "BSM2_66"
  Data Type Conversion58/1 -> [bsm_yaw_rate_2]  "BSM2_57"
  Data Type Conversion59/1 -> [bsm_brk_status_2]  "BSM2_58"
  Data Type Conversion6/1 -> [N_a_2]  "BSM2_16"
  Data Type Conversion60/1 -> [wheel_brk_unavailable_2]  "BSM2_59"
  Data Type Conversion61/1 -> [traction_contr_state_2]  "BSM2_60"
  Data Type Conversion62/1 -> [anti_lock_brk_status_2]  "BSM2_61"
  Data Type Conversion63/1 -> [stability_control_status_2]  "BSM2_62"
  Data Type Conversion64/1 -> [brk_boost_enum_2]  "BSM2_63"
  Data Type Conversion65/1 -> [auxi_brk_status_enum_2]  "BSM2_64"
  Data Type Conversion66/1 -> [veh_height_2]  "BSM2_65"
  Data Type Conversion7/1 -> [E_a_2]  "BSM2_17"
  Data Type Conversion78/1 -> [user_def_1_2]  "BSM2_67"
  Data Type Conversion79/1 -> [user_def_2_2]  "BSM2_68"
  Data Type Conversion8/1 -> [D_a_2]  "BSM2_18"
  Data Type Conversion80/1 -> [user_def_3_2]  "BSM2_69"
  Data Type Conversion81/1 -> [user_def_4_2]  "BSM2_70"
  Data Type Conversion82/1 -> [user_def_5_2]  "BSM2_71"
  Data Type Conversion9/1 -> [grp_id_2]  "BSM2_19"
  Data Type Conversion68/1 -> Data Type Conversion81/1
  Data Type Conversion69/1 -> Data Type Conversion79/1
  Data Type Conversion67/1 -> Data Type Conversion82/1
  Data Type Conversion70/1 -> Data Type Conversion80/1
  Data Type Conversion71/1 -> Data Type Conversion78/1

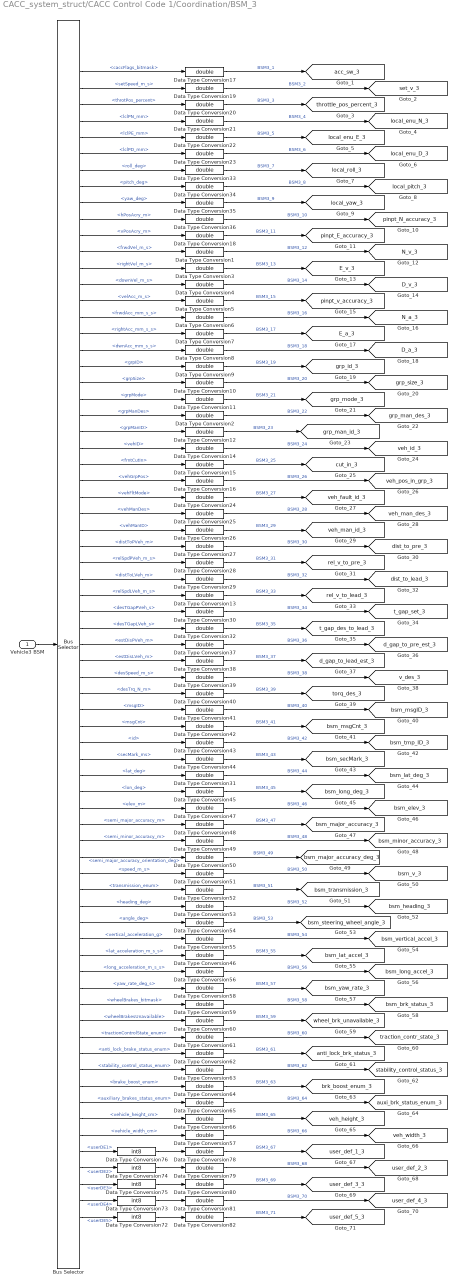
== system CACC_system_struct/CACC Control Code 1/Coordination/BSM_3 ==
  Vehicle3 BSM : Inport
  Bus Selector : BusSelector  OutputSignals=caccFlags_bitmask,setSpeed_m_s,throtPos_percent,lclPN_mm,lclPE_mm,lclPD_mm,roll_deg,pitch_deg,yaw_deg,hPosAcry_m,vPosAcry_m,frwdVel_m_s,rightVel_m_s,downVel_m_s,velAcc_m_s,frwdAcc_mm_s_s,rightAcc_mm_s_s,dwnAcc_mm_s_s,grpID,grpSize,grpMode,grpManDes,grpManID,vehID,frntCutIn,vehGrpPos,vehFltMode,vehManDes,vehManID,distToPVeh_m,relSpdPVeh_m_s,distToLVeh_m,relSpdLVeh_m_s,desTGapPVeh_s,desTGapLVeh_s,estDisPVeh_m,estDisLVeh_m,desSpeed_m_s,desTrq_N_m,msgID,msgCnt,id,secMark_ms,lat_deg,lon_deg,elev_m,semi_major_accuracy_m,semi_minor_accuracy_m,semi_major_accuracy_orientation_deg,speed_m_s,transmission_enum,heading_deg,angle_deg,vertical_acceleration_g,lat_acceleration_m_s_s,long_acceleration_m_s_s,yaw_rate_deg_s,wheelBrakes_bitmask,wheelBrakesUnavailable,tractionControlState_enum,anti_lock_brake_status_enum,stability_control_status_enum,brake_boost_enum,auxiliary_brakes_status_enum,vehicle_height_cm,vehicle_width_cm,userDE1,userDE2,userDE3,userDE4,userDE5
  Data Type Conversion{1..66,78..82} (71 alike) : DataTypeConversion  OutMin=[0]  OutMax=[5]  OutDataTypeStr=double
  Data Type Conversion{72..76} (5 alike) : DataTypeConversion  OutMin=[-128]  OutMax=[127]  OutDataTypeStr=int8  ConvertRealWorld=Stored Integer (SI)
  tag scope: D_a_3=global, D_v_3=global, E_a_3=global, E_v_3=global, N_a_3=global, N_v_3=global, acc_sw_3=global, anti_lock_brk_status_3=global, auxi_brk_status_enum_3=global, brk_boost_enum_3=global, bsm_brk_status_3=global, bsm_elev_3=global, bsm_heading_3=global, bsm_lat_accel_3=global, bsm_lat_deg_3=global, bsm_long_accel_3=global, bsm_long_deg_3=global, bsm_major_accuracy_3=global, bsm_major_accuracy_deg_3=global, bsm_minor_accuracy_3=global, bsm_msgCnt_3=global, bsm_msgID_3=global, bsm_secMark_3=global, bsm_steering_wheel_angle_3=global, bsm_tmp_ID_3=global, bsm_transmission_3=global, bsm_v_3=global, bsm_vertical_accel_3=global, bsm_yaw_rate_3=global, cut_in_3=global, d_gap_to_lead_est_3=global, d_gap_to_pre_est_3=global, dist_to_lead_3=global, dist_to_pre_3=global, grp_id_3=global, grp_man_des_3=global, grp_man_id_3=global, grp_mode_3=global, grp_size_3=global, local_enu_D_3=global, local_enu_E_3=global, local_enu_N_3=global, local_pitch_3=global, local_roll_3=global, local_yaw_3=global, pinpt_E_accuracy_3=global, pinpt_N_accuracy_3=global, pinpt_v_accuracy_3=global, rel_v_to_lead_3=global, rel_v_to_pre_3=global, set_v_3=global, stability_control_status_3=global, t_gap_des_to_lead_3=global, t_gap_set_3=global, throttle_pos_percent_3=global, torq_des_3=global, traction_contr_state_3=global, user_def_1_3=global, user_def_2_3=global, user_def_3_3=global, user_def_4_3=global, user_def_5_3=global, v_des_3=global, veh_fault_id_3=global, veh_height_3=global, veh_id_3=global, veh_man_des_3=global, veh_man_id_3=global, veh_pos_in_grp_3=global, veh_width_3=global, wheel_brk_unavailable_3=global
  wires:
  Vehicle3 BSM/1 -> Bus Selector/1
  Bus Selector/34 -> Data Type Conversion30/1  "<desTGapPVeh_s>"
  Bus Selector/33 -> Data Type Conversion13/1  "<relSpdLVeh_m_s>"
  Bus Selector/2 -> Data Type Conversion19/1  "<setSpeed_m_s>"
  Bus Selector/1 -> Data Type Conversion17/1  "<caccFlags_bitmask>"
  Bus Selector/7 -> Data Type Conversion33/1  "<roll_deg>"
  Bus Selector/3 -> Data Type Conversion20/1  "<throtPos_percent>"
  Bus Selector/9 -> Data Type Conversion35/1  "<yaw_deg>"
  Bus Selector/8 -> Data Type Conversion34/1  "<pitch_deg>"
  Bus Selector/11 -> Data Type Conversion18/1  "<vPosAcry_m>"
  Bus Selector/10 -> Data Type Conversion36/1  "<hPosAcry_m>"
  Bus Selector/13 -> Data Type Conversion3/1  "<rightVel_m_s>"
  Bus Selector/12 -> Data Type Conversion1/1  "<frwdVel_m_s>"
  Bus Selector/15 -> Data Type Conversion5/1  "<velAcc_m_s>"
  Bus Selector/14 -> Data Type Conversion4/1  "<downVel_m_s>"
  Bus Selector/17 -> Data Type Conversion7/1  "<rightAcc_mm_s_s>"
  Bus Selector/16 -> Data Type Conversion6/1  "<frwdAcc_mm_s_s>"
  Bus Selector/19 -> Data Type Conversion9/1  "<grpID>"
  Bus Selector/18 -> Data Type Conversion8/1  "<dwnAcc_mm_s_s>"
  Bus Selector/21 -> Data Type Conversion11/1  "<grpMode>"
  Bus Selector/20 -> Data Type Conversion10/1  "<grpSize>"
  Bus Selector/22 -> Data Type Conversion2/1  "<grpManDes>"
  Bus Selector/25 -> Data Type Conversion15/1  "<frntCutIn>"
  Bus Selector/24 -> Data Type Conversion14/1  "<vehID>"
  Bus Selector/27 -> Data Type Conversion24/1  "<vehFltMode>"
  Bus Selector/26 -> Data Type Conversion16/1  "<vehGrpPos>"
  Bus Selector/30 -> Data Type Conversion27/1  "<distToPVeh_m>"
  Bus Selector/29 -> Data Type Conversion26/1  "<vehManID>"
  Bus Selector/32 -> Data Type Conversion29/1  "<distToLVeh_m>"
  Bus Selector/36 -> Data Type Conversion37/1  "<estDisPVeh_m>"
  Bus Selector/35 -> Data Type Conversion32/1  "<desTGapLVeh_s>"
  Bus Selector/38 -> Data Type Conversion39/1  "<desSpeed_m_s>"
  Bus Selector/37 -> Data Type Conversion38/1  "<estDisLVeh_m>"
  Bus Selector/40 -> Data Type Conversion41/1  "<msgID>"
  Bus Selector/39 -> Data Type Conversion40/1  "<desTrq_N_m>"
  Bus Selector/42 -> Data Type Conversion43/1  "<id>"
  Bus Selector/41 -> Data Type Conversion42/1  "<msgCnt>"
  Bus Selector/44 -> Data Type Conversion31/1  "<lat_deg>"
  Bus Selector/43 -> Data Type Conversion44/1  "<secMark_ms>"
  Bus Selector/46 -> Data Type Conversion47/1  "<elev_m>"
  Bus Selector/45 -> Data Type Conversion45/1  "<lon_deg>"
  Bus Selector/48 -> Data Type Conversion49/1  "<semi_minor_accuracy_m>"
  Bus Selector/47 -> Data Type Conversion48/1  "<semi_major_accuracy_m>"
  Bus Selector/50 -> Data Type Conversion51/1  "<speed_m_s>"
  Bus Selector/49 -> Data Type Conversion50/1  "<semi_major_accuracy_orientation_deg>"
  Bus Selector/52 -> Data Type Conversion53/1  "<heading_deg>"
  Bus Selector/51 -> Data Type Conversion52/1  "<transmission_enum>"
  Bus Selector/54 -> Data Type Conversion55/1  "<vertical_acceleration_g>"
  Bus Selector/53 -> Data Type Conversion54/1  "<angle_deg>"
  Bus Selector/56 -> Data Type Conversion56/1  "<long_acceleration_m_s_s>"
  Bus Selector/55 -> Data Type Conversion46/1  "<lat_acceleration_m_s_s>"
  Bus Selector/58 -> Data Type Conversion59/1  "<wheelBrakes_bitmask>"
  Bus Selector/57 -> Data Type Conversion58/1  "<yaw_rate_deg_s>"
  Bus Selector/60 -> Data Type Conversion61/1  "<tractionControlState_enum>"
  Bus Selector/59 -> Data Type Conversion60/1  "<wheelBrakesUnavailable>"
  Bus Selector/62 -> Data Type Conversion63/1  "<stability_control_status_enum>"
  Bus Selector/61 -> Data Type Conversion62/1  "<anti_lock_brake_status_enum>"
  Bus Selector/64 -> Data Type Conversion65/1  "<auxiliary_brakes_status_enum>"
  Bus Selector/63 -> Data Type Conversion64/1  "<brake_boost_enum>"
  Bus Selector/66 -> Data Type Conversion57/1  "<vehicle_width_cm>"
  Bus Selector/65 -> Data Type Conversion66/1  "<vehicle_height_cm>"
  Bus Selector/4 -> Data Type Conversion21/1  "<lclPN_mm>"
  Bus Selector/5 -> Data Type Conversion22/1  "<lclPE_mm>"
  Bus Selector/6 -> Data Type Conversion23/1  "<lclPD_mm>"
  Bus Selector/23 -> Data Type Conversion12/1  "<grpManID>"
  Bus Selector/28 -> Data Type Conversion25/1  "<vehManDes>"
  Bus Selector/31 -> Data Type Conversion28/1  "<relSpdPVeh_m_s>"
  Bus Selector/67 -> Data Type Conversion76/1  "<userDE1>"
  Bus Selector/68 -> Data Type Conversion74/1  "<userDE2>"
  Bus Selector/69 -> Data Type Conversion75/1  "<userDE3>"
  Bus Selector/70 -> Data Type Conversion73/1  "<userDE4>"
  Bus Selector/71 -> Data Type Conversion72/1  "<userDE5>"
  Data Type Conversion38/1 -> [d_gap_to_lead_est_3]  "BSM3_37"
  Data Type Conversion17/1 -> [acc_sw_3]  "BSM3_1"
  Data Type Conversion16/1 -> [veh_pos_in_grp_3]  "BSM3_26"
  Data Type Conversion6/1 -> [N_a_3]  "BSM3_16"
  Data Type Conversion50/1 -> [bsm_major_accuracy_deg_3]  "BSM3_49"
  Data Type Conversion36/1 -> [pinpt_N_accuracy_3]  "BSM3_10"
  Data Type Conversion14/1 -> [veh_id_3]  "BSM3_24"
  Data Type Conversion82/1 -> [user_def_5_3]  "BSM3_71"
  Data Type Conversion54/1 -> [bsm_steering_wheel_angle_3]  "BSM3_53"
  Data Type Conversion12/1 -> [grp_man_id_3]  "BSM3_23"
  Data Type Conversion79/1 -> [user_def_2_3]  "BSM3_68"
  Data Type Conversion7/1 -> [E_a_3]  "BSM3_17"
  Data Type Conversion62/1 -> [anti_lock_brk_status_3]  "BSM3_61"
  Data Type Conversion49/1 -> [bsm_minor_accuracy_3]  "BSM3_48"
  Data Type Conversion20/1 -> [throttle_pos_percent_3]  "BSM3_3"
  Data Type Conversion59/1 -> [bsm_brk_status_3]  "BSM3_58"
  Data Type Conversion47/1 -> [bsm_elev_3]  "BSM3_46"
  Data Type Conversion48/1 -> [bsm_major_accuracy_3]  "BSM3_47"
  Data Type Conversion2/1 -> [grp_man_des_3]  "BSM3_22"
  Data Type Conversion24/1 -> [veh_fault_id_3]  "BSM3_27"
  Data Type Conversion30/1 -> [t_gap_set_3]  "BSM3_34"
  Data Type Conversion45/1 -> [bsm_long_deg_3]  "BSM3_45"
  Data Type Conversion13/1 -> [rel_v_to_lead_3]  "BSM3_33"
  Data Type Conversion78/1 -> [user_def_1_3]  "BSM3_67"
  Data Type Conversion9/1 -> [grp_id_3]  "BSM3_19"
  Data Type Conversion41/1 -> [bsm_msgID_3]  "BSM3_40"
  Data Type Conversion26/1 -> [veh_man_id_3]  "BSM3_29"
  Data Type Conversion40/1 -> [torq_des_3]  "BSM3_39"
  Data Type Conversion27/1 -> [dist_to_pre_3]  "BSM3_30"
  Data Type Conversion32/1 -> [t_gap_des_to_lead_3]  "BSM3_35"
  Data Type Conversion60/1 -> [wheel_brk_unavailable_3]  "BSM3_59"
  Data Type Conversion35/1 -> [local_yaw_3]  "BSM3_9"
  Data Type Conversion39/1 -> [v_des_3]  "BSM3_38"
  Data Type Conversion63/1 -> [stability_control_status_3]  "BSM3_62"
  Data Type Conversion23/1 -> [local_enu_D_3]  "BSM3_6"
  Data Type Conversion56/1 -> [bsm_long_accel_3]  "BSM3_56"
  Data Type Conversion65/1 -> [auxi_brk_status_enum_3]  "BSM3_64"
  Data Type Conversion53/1 -> [bsm_heading_3]  "BSM3_52"
  Data Type Conversion10/1 -> [grp_size_3]  "BSM3_20"
  Data Type Conversion19/1 -> [set_v_3]  "BSM3_2"
  Data Type Conversion64/1 -> [brk_boost_enum_3]  "BSM3_63"
  Data Type Conversion37/1 -> [d_gap_to_pre_est_3]  "BSM3_36"
  Data Type Conversion11/1 -> [grp_mode_3]  "BSM3_21"
  Data Type Conversion66/1 -> [veh_height_3]  "BSM3_65"
  Data Type Conversion80/1 -> [user_def_3_3]  "BSM3_69"
  Data Type Conversion34/1 -> [local_pitch_3]  "BSM3_8"
  Data Type Conversion5/1 -> [pinpt_v_accuracy_3]  "BSM3_15"
  Data Type Conversion51/1 -> [bsm_v_3]  "BSM3_50"
  Data Type Conversion33/1 -> [local_roll_3]  "BSM3_7"
  Data Type Conversion1/1 -> [N_v_3]  "BSM3_12"
  Data Type Conversion46/1 -> [bsm_lat_accel_3]  "BSM3_55"
  Data Type Conversion55/1 -> [bsm_vertical_accel_3]  "BSM3_54"
  Data Type Conversion52/1 -> [bsm_transmission_3]  "BSM3_51"
  Data Type Conversion28/1 -> [rel_v_to_pre_3]  "BSM3_31"
  Data Type Conversion81/1 -> [user_def_4_3]  "BSM3_70"
  Data Type Conversion57/1 -> [veh_width_3]  "BSM3_66"
  Data Type Conversion25/1 -> [veh_man_des_3]  "BSM3_28"
  Data Type Conversion8/1 -> [D_a_3]  "BSM3_18"
  Data Type Conversion42/1 -> [bsm_msgCnt_3]  "BSM3_41"
  Data Type Conversion29/1 -> [dist_to_lead_3]  "BSM3_32"
  Data Type Conversion43/1 -> [bsm_tmp_ID_3]  "BSM3_42"
  Data Type Conversion18/1 -> [pinpt_E_accuracy_3]  "BSM3_11"
  Data Type Conversion3/1 -> [E_v_3]  "BSM3_13"
  Data Type Conversion44/1 -> [bsm_secMark_3]  "BSM3_43"
  Data Type Conversion22/1 -> [local_enu_E_3]  "BSM3_5"
  Data Type Conversion15/1 -> [cut_in_3]  "BSM3_25"
  Data Type Conversion21/1 -> [local_enu_N_3]  "BSM3_4"
  Data Type Conversion58/1 -> [bsm_yaw_rate_3]  "BSM3_57"
  Data Type Conversion61/1 -> [traction_contr_state_3]  "BSM3_60"
  Data Type Conversion31/1 -> [bsm_lat_deg_3]  "BSM3_44"
  Data Type Conversion4/1 -> [D_v_3]  "BSM3_14"
  Data Type Conversion76/1 -> Data Type Conversion78/1
  Data Type Conversion73/1 -> Data Type Conversion81/1
  Data Type Conversion74/1 -> Data Type Conversion79/1
  Data Type Conversion75/1 -> Data Type Conversion80/1
  Data Type Conversion72/1 -> Data Type Conversion82/1
